simulink model "multipathfadig"  (R2024b)
settings: Solver=VariableStepAuto  StartTime=0.0  StopTime=10.0  RelTol=1e-3
undefined symbols (not defined in the file): doppler, magnitude
libraries: commchan3 x2, dspmathops x2, commrandsrc3 x1, commdigbbndpm3 x1
settings Model: Creator=ahari  LastModifiedBy=ahari

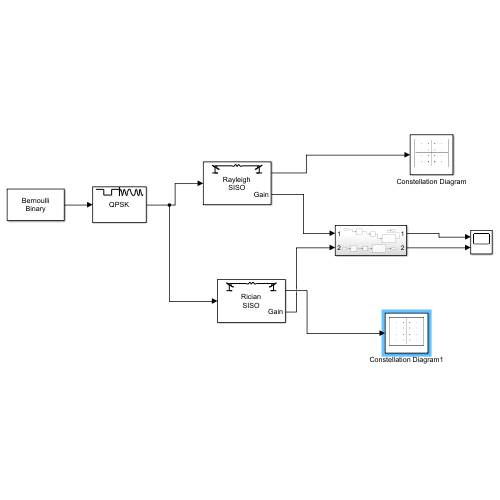
[thumbnail: Simulink's stored preview of the top-level diagram]
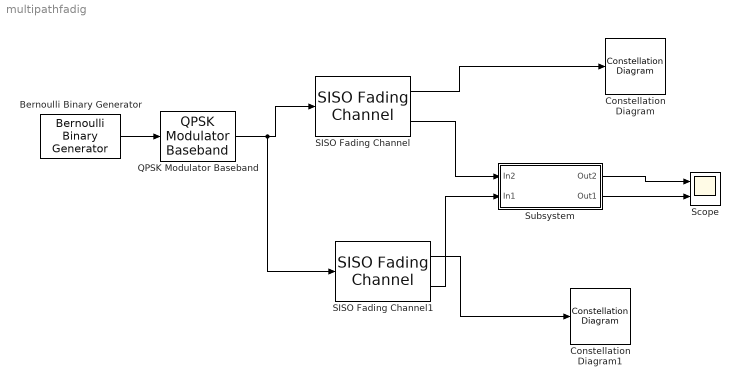
== system multipathfadig ==
  Bernoulli Binary Generator : commrandsrc3/Bernoulli Binary Generator  ProbabilityOfZero=0.5  SeedSource=Auto  Seed=61  SampleTime=1e-6  SamplesPerFrame=1000  OutputDataType=double  SimulateUsing=Interpreted execution
  Constellation Diagram : ConstellationDiagram  WindowPosition=[382.000000,84.000000,600.000000,600.000000,]  ScopeFrameLocation=window  DefaultConfigurationName=comm.scopes.ConstellationDiagramBlockCfg
  Constellation Diagram1 : ConstellationDiagram  WindowPosition=[382.000000,84.000000,600.000000,600.000000,]  ScopeFrameLocation=window  DefaultConfigurationName=comm.scopes.ConstellationDiagramBlockCfg
  QPSK Modulator Baseband : commdigbbndpm3/QPSK Modulator Baseband  InType=Integer  Enc=Gray  Ph=pi/4  outDtype=double  outWordLen=16  outUDDataType=sfix(16)  outFracLenMode=Best precision  outFracLen=15  outDataTypeStr=double  outLastDataTypeStr=double
  SISO Fading Channel : commchan3/SISO Fading Channel  InheritSampleRate=on  SampleRate=1  PathDelays=[0 0.2e-7 0.4e-7 0.8e-7]  AveragePathGains=[0 -3 -6 -9]  NormalizePathGains=on  FadingDistribution=Rayleigh  KFactor=3  DirectPathDopplerShift=0  DirectPathInitialPhase=0  MaximumDopplerShift=200  DopplerSpectrum=doppler('Jakes')  RandomStream=mt19937ar with seed  Seed=73  PathGainsOutputPort=on  ChannelFilterDelayOutputPort=off  SimulateUsing=Interpreted execution  Visualization=Off  PathsForDopplerDisplay=1  SamplesToDisplay=25%
  SISO Fading Channel1 : commchan3/SISO Fading Channel  InheritSampleRate=on  SampleRate=1  PathDelays=[0, 0.2e-7, 0.4e-7, 0.8e-7]  AveragePathGains=[0, -3, -6, -9]  NormalizePathGains=on  FadingDistribution=Rician  KFactor=10  DirectPathDopplerShift=100  DirectPathInitialPhase=0  MaximumDopplerShift=200  DopplerSpectrum=doppler('Jakes')  RandomStream=mt19937ar with seed  Seed=73  PathGainsOutputPort=on  ChannelFilterDelayOutputPort=off  SimulateUsing=Interpreted execution  Visualization=Off  PathsForDopplerDisplay=1  SamplesToDisplay=25%
  Scope : Scope  NumInputPorts=2
  Subsystem : Subsystem
  wires:
  Bernoulli Binary Generator/1 -> QPSK Modulator Baseband/1
  QPSK Modulator Baseband/1 -> SISO Fading Channel1/1, SISO Fading Channel/1
  SISO Fading Channel/1 -> Constellation Diagram/1
  SISO Fading Channel1/1 -> Constellation Diagram1/1
  Subsystem/1(Out2) -> Scope/1
  Subsystem/2(Out1) -> Scope/2
  SISO Fading Channel/2 -> Subsystem/1(In2)
  SISO Fading Channel1/2 -> Subsystem/2(In1)

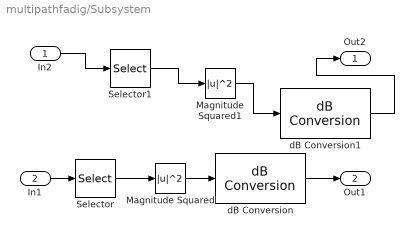
== system multipathfadig/Subsystem ==
  In2 : Inport
  In1 : Inport  Port=2
  Magnitude Squared : Math  Operator=magnitude^2
  Magnitude Squared1 : Math  Operator=magnitude^2
  Selector : Selector  NumberOfDimensions=2  InputPortWidth=3  IndexOptions=Select all,Index vector (dialog)  Indices=[1 3],1  OutputSizes=1,1
  Selector1 : Selector  NumberOfDimensions=2  InputPortWidth=3  IndexOptions=Select all,Index vector (dialog)  Indices=[1 3],1  OutputSizes=1,1
  dB Conversion : dspmathops/dB Conversion  dBtype=dB  intype=Power  R=1  fuzz=off
      settings: LibrarySourceBlock=commutil2/dB Conversion
  dB Conversion1 : dspmathops/dB Conversion  dBtype=dB  intype=Power  R=1  fuzz=off
      settings: LibrarySourceBlock=commutil2/dB Conversion
  Out2 : Outport
  Out1 : Outport  Port=2
  wires:
  In1/1 -> Selector/1
  Selector/1 -> Magnitude Squared/1
  Magnitude Squared/1 -> dB Conversion/1
  dB Conversion/1 -> Out1/1
  In2/1 -> Selector1/1
  Selector1/1 -> Magnitude Squared1/1
  Magnitude Squared1/1 -> dB Conversion1/1
  dB Conversion1/1 -> Out2/1
